simulink model "lectura_presion"  (R2022a)
settings: Solver=VariableStepAuto  StartTime=0.0  StopTime=inf  RelTol=1e-3
values from neighbouring files (symbols this model uses):
  outputmax = 16777216 * (outputmax / 100.0) + 0.5    (= 15099494.9)    [control.m]    (also in params.mat)
  outputmin = 16777216 * (outputmin / 100.0) + 0.5    (= 1677722.1)    [control.m]    (also in params.mat)
  pmax = 25    [control.m]    (also in params.mat)
  pmin = 0    [control.m]    (also in params.mat)
libraries: instrumentseriallib x2, hdlsllib x1
settings Model: Creator=Ponchito  LastModifiedBy=Ponchito

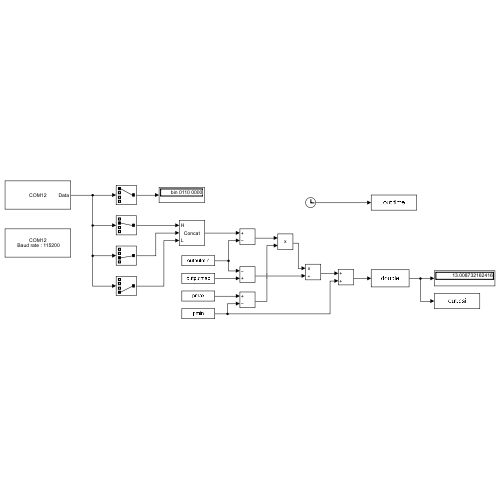
[thumbnail: Simulink's stored preview of the top-level diagram]
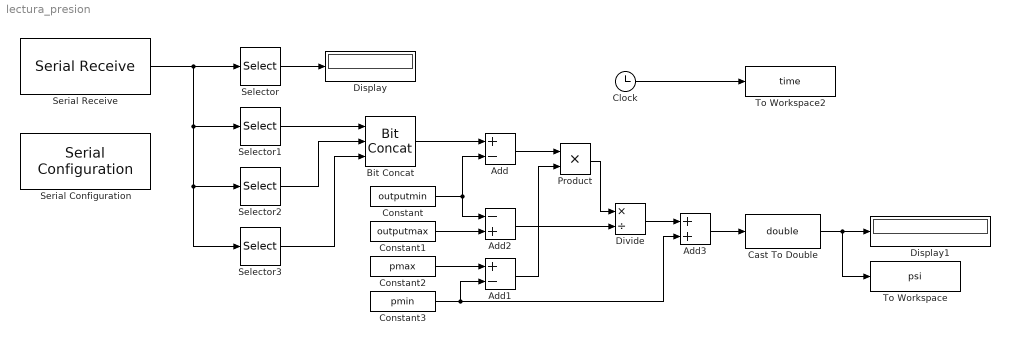
== system lectura_presion ==
  Add : Sum  Inputs=+-
  Add1 : Sum  Inputs=+-
  Add2 : Sum  Inputs=-+
  Add3 : Sum
  Bit Concat : hdlsllib/Logic and Bit Operations/Bit Concat  numInputs=3
  Cast To Double : DataTypeConversion  OutDataTypeStr=double  SaturateOnIntegerOverflow=off  RndMeth=Floor
  Clock : Clock
  Constant : Constant  Value=outputmin
  Constant1 : Constant  Value=outputmax
  Constant2 : Constant  Value=pmax
  Constant3 : Constant  Value=pmin
  Display : Display
      settings: Format=binary (Stored Integer)
  Display1 : Display
  Divide : Product  Inputs=*/
  Product : Product
  Selector : Selector  InputPortWidth=4  IndexOptions=Index vector (dialog)  Indices=1  OutputSizes=1
  Selector1 : Selector  InputPortWidth=4  IndexOptions=Index vector (dialog)  Indices=2  OutputSizes=1
  Selector2 : Selector  InputPortWidth=4  IndexOptions=Index vector (dialog)  Indices=3  OutputSizes=1
  Selector3 : Selector  InputPortWidth=4  IndexOptions=Index vector (dialog)  Indices=4  OutputSizes=1
  Serial Configuration : instrumentseriallib/Serial Configuration  Priority=-200000  PortSel=COM12  Port=COM12  ComPort=COM12  BaudRate=115200  DataBits=8  Parity=none  StopBits=1  ByteOrder=little-endian  FlowControl=none  Timeout=10  SimulateUsing=Interpreted execution  BlockInModel=on  aMode=1
      settings: SourceProductBaseCode=OT,IC,MT
  Serial Receive : instrumentseriallib/Serial Receive  Priority=1  PortSel=COM12  Port=COM12  ComPort=COM12  DataType=uint8  SaveDataType=uint8  ToggleHeader=off  Header=[]  ToggleTerminator=off  Terminator=<none>  CustomTerminator=[]  InputFormat=Column major  ToggleDataSize=on  DataSize=[1 4]  EnableBlockingMode=on  ActionDataUnavailable=Output last received value  ActionWhenDataUnavailable=Output last received value  CustomValue=0  SampleTime=0.1  SimulateUsing=Interpreted execution  BlockInModel=on  aMode=1
      settings: SourceProductBaseCode=OT,IC,MT
  To Workspace : ToWorkspace  VariableName=psi  SaveFormat=Timeseries  SampleTime=-1
  To Workspace2 : ToWorkspace  VariableName=time  SampleTime=-1
  wires:
  Serial Receive/1 -> Selector3/1, Selector2/1, Selector1/1, Selector/1
  Selector/1 -> Display/1
  Selector1/1 -> Bit Concat/1
  Selector2/1 -> Bit Concat/2
  Selector3/1 -> Bit Concat/3
  Bit Concat/1 -> Add/1
  Constant/1 -> Add2/1, Add/2
  Constant2/1 -> Add1/1
  Constant3/1 -> Add3/2, Add1/2
  Add/1 -> Product/1
  Add1/1 -> Product/2
  Constant1/1 -> Add2/2
  Product/1 -> Divide/1
  Add2/1 -> Divide/2
  Divide/1 -> Add3/1
  Clock/1 -> To Workspace2/1
  Add3/1 -> Cast To Double/1
  Cast To Double/1 -> Display1/1, To Workspace/1
